simulink library "SensorLibrary"  (R2017a)
settings: Solver=VariableStepAuto  StartTime=0.0  StopTime=10.0  RelTol=1e-3
settings Model: Creator=ptracton  LastModifiedBy=ptracton

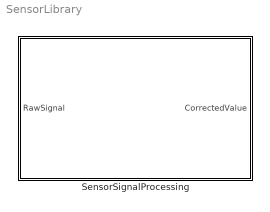
== system SensorLibrary ==
  SensorSignalProcessing : Subsystem  mask{Slope=20, Offset=-20}
      mask DialogControl DescTextVar Prompt: This block allows you to add a slope and offset to a raw signal value
      mask DialogControl Control3 Prompt: Slope
      mask DialogControl Control2 Prompt: Offset

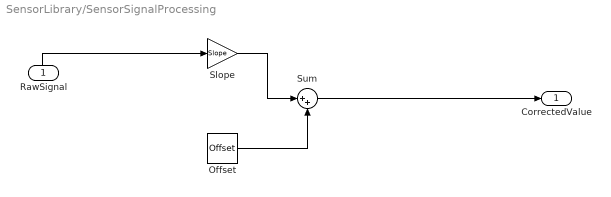
== system SensorLibrary/SensorSignalProcessing ==
  RawSignal : Inport
  Offset : Constant  Value=Offset
  Slope : Gain  Gain=Slope
  Sum : Sum  Inputs=|++
  CorrectedValue : Outport
  wires:
  Offset/1 -> Sum/2
  RawSignal/1 -> Slope/1
  Sum/1 -> CorrectedValue/1
  Slope/1 -> Sum/1
